simulink model "empirical_cell_twaice_balancing"  (R2024b)
settings: Solver=FixedStepAuto  StartTime=0.0  StopTime=inf  FixedStep=1  RelTol=1e-3
values from neighbouring files (symbols this model uses):
  act = 1    [RunMe_TWAICE_Cell_Model_Farasis_P75_75Ah_v8_1_3.m]
  lic_no = fin_convert(Prod_lic)    [RunMe_TWAICE_Cell_Model_Farasis_P75_75Ah_v8_1_3.m]
  Ts = 1    [RunMe_TWAICE_Cell_Model_Farasis_P75_75Ah_v8_1_3.m]
undefined symbols (not defined in the file or in its folder): DWORK0, DWORK1, DWORK10, DWORK11, DWORK12, DWORK13, DWORK14, DWORK15, DWORK16, DWORK17, DWORK18, DWORK19, DWORK2, DWORK20, DWORK22, DWORK23, DWORK24, DWORK25, DWORK26, DWORK27, DWORK28, DWORK29, DWORK3, DWORK30, DWORK31, DWORK32, DWORK33, DWORK34, DWORK35, DWORK36, DWORK4, DWORK5, DWORK6, DWORK7, DWORK8, DWORK9, SOHc_init, SOHr_init
libraries: fl_lib x73, nesl_utility x32, ee_lib x8
(part 1 of 4)
settings Model: PacingRate=60  Creator=CARSCH  LastModifiedBy=CARSCH
settings DebuggingCC: AlgebraicLoopMsg=none

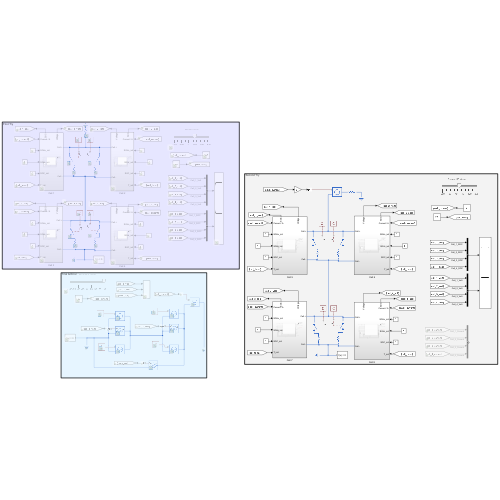
[thumbnail: Simulink's stored preview of the top-level diagram]
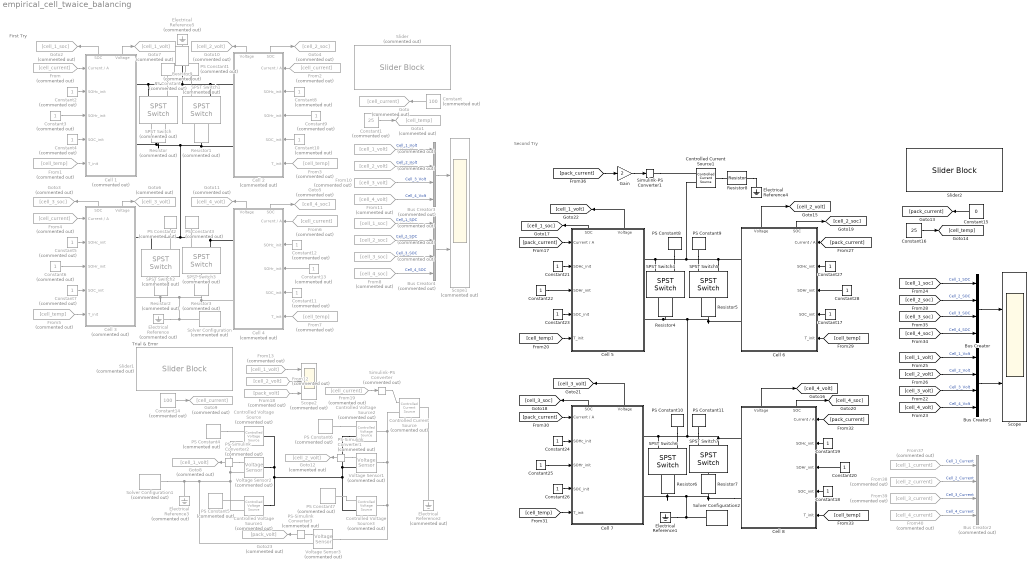
== system empirical_cell_twaice_balancing ==
  note: Trial & Error
  note: First Try
  note: Second Try
  Bus Creator : BusCreator  Inputs=4
  Bus Creator1 : BusCreator  Inputs=4
  Bus Creator2 : BusCreator  Commented=on  Inputs=4
  Bus Creator3 : BusCreator  Commented=on  Inputs=4
  Bus Creator4 : BusCreator  Commented=on  Inputs=4
  Cell 1 : Subsystem  Commented=on
      settings: PortSchema="{\"entries\":[{\"content\":{\"sides\":[{\"content\":{\"connectorIds\":[\"In1\",\"In2\",\"In3\",\"In4\",\"In5\"]},\"type\":\"ConnectorPlacement.EquallySpacedRectSide\",\"uuid\":\"39b6e759-d3e5-472a-9e81-7460229c4a62\"},{\"content\":{\"connectorIds\":[\"RConn1\",\"RConn2\"],\"side\":\"RIGHT\"},\"type\":\"ConnectorPlacement.EquallySpacedRectSide\",\"uuid\":\"f7fe5ccd-0242-4e3e-8253-e5b9b00b3385\"},{\"content\":{\"connectorIds\":[\"Out1\",\"Out2\"],\"side\":\"TOP\"},\"type\":\"ConnectorPlacement.EquallySpacedRectSide\",\"uuid\":\"deea17ee-3044-4fb2-b027-954681f0d31b\"}]},\"type\":\"ConnectorPlacement.EquallySpacedConnector\",\"uuid\":\"64bf650a-96e4-4191-8eb1-250115cba883\"}],\"packageUris\":[\"http://schema.mathworks.com/mf0/Connector/R2020b\"],\"version\":\"1.0\"}"
  Cell 2 : Subsystem  Commented=on
      settings: PortSchema="{\"entries\":[{\"content\":{\"sides\":[{\"content\":{\"connectorIds\":[\"In1\",\"In2\",\"In3\",\"In4\",\"In5\"]},\"type\":\"ConnectorPlacement.EquallySpacedRectSide\",\"uuid\":\"d8dd5e7d-9ddf-43d8-85ce-2acbe04dd73f\"},{\"content\":{\"connectorIds\":[\"RConn1\",\"RConn2\"],\"side\":\"RIGHT\"},\"type\":\"ConnectorPlacement.EquallySpacedRectSide\",\"uuid\":\"568b7dc0-f917-4967-8cc2-cd04b3e2240a\"},{\"content\":{\"connectorIds\":[\"Out1\",\"Out2\"],\"side\":\"TOP\"},\"type\":\"ConnectorPlacement.EquallySpacedRectSide\",\"uuid\":\"9700caac-c62d-4472-a735-ae999ee4f2e3\"}]},\"type\":\"ConnectorPlacement.EquallySpacedConnector\",\"uuid\":\"46beb2be-287e-49be-b6c7-ffcf4a8dc46d\"}],\"packageUris\":[\"http://schema.mathworks.com/mf0/Connector/R2020b\"],\"version\":\"1.0\"}"
  Cell 3 : Subsystem  Commented=on
      settings: PortSchema="{\"entries\":[{\"content\":{\"sides\":[{\"content\":{\"connectorIds\":[\"In1\",\"In2\",\"In3\",\"In4\",\"In5\"]},\"type\":\"ConnectorPlacement.EquallySpacedRectSide\",\"uuid\":\"d8dd5e7d-9ddf-43d8-85ce-2acbe04dd73f\"},{\"content\":{\"connectorIds\":[\"RConn1\",\"RConn2\"],\"side\":\"RIGHT\"},\"type\":\"ConnectorPlacement.EquallySpacedRectSide\",\"uuid\":\"568b7dc0-f917-4967-8cc2-cd04b3e2240a\"},{\"content\":{\"connectorIds\":[\"Out1\",\"Out2\"],\"side\":\"TOP\"},\"type\":\"ConnectorPlacement.EquallySpacedRectSide\",\"uuid\":\"9700caac-c62d-4472-a735-ae999ee4f2e3\"}]},\"type\":\"ConnectorPlacement.EquallySpacedConnector\",\"uuid\":\"46beb2be-287e-49be-b6c7-ffcf4a8dc46d\"}],\"packageUris\":[\"http://schema.mathworks.com/mf0/Connector/R2020b\"],\"version\":\"1.0\"}"
  Cell 4 : Subsystem  Commented=on
      settings: PortSchema="{\"entries\":[{\"content\":{\"sides\":[{\"content\":{\"connectorIds\":[\"In1\",\"In2\",\"In3\",\"In4\",\"In5\"]},\"type\":\"ConnectorPlacement.EquallySpacedRectSide\",\"uuid\":\"d8dd5e7d-9ddf-43d8-85ce-2acbe04dd73f\"},{\"content\":{\"connectorIds\":[\"RConn1\",\"RConn2\"],\"side\":\"RIGHT\"},\"type\":\"ConnectorPlacement.EquallySpacedRectSide\",\"uuid\":\"568b7dc0-f917-4967-8cc2-cd04b3e2240a\"},{\"content\":{\"connectorIds\":[\"Out1\",\"Out2\"],\"side\":\"TOP\"},\"type\":\"ConnectorPlacement.EquallySpacedRectSide\",\"uuid\":\"9700caac-c62d-4472-a735-ae999ee4f2e3\"}]},\"type\":\"ConnectorPlacement.EquallySpacedConnector\",\"uuid\":\"46beb2be-287e-49be-b6c7-ffcf4a8dc46d\"}],\"packageUris\":[\"http://schema.mathworks.com/mf0/Connector/R2020b\"],\"version\":\"1.0\"}"
  Cell 5 : Subsystem
      settings: PortSchema="{\"entries\":[{\"content\":{\"sides\":[{\"content\":{\"connectorIds\":[\"In1\",\"In2\",\"In3\",\"In4\",\"In5\"]},\"type\":\"ConnectorPlacement.EquallySpacedRectSide\",\"uuid\":\"39b6e759-d3e5-472a-9e81-7460229c4a62\"},{\"content\":{\"connectorIds\":[\"RConn1\",\"RConn2\"],\"side\":\"RIGHT\"},\"type\":\"ConnectorPlacement.EquallySpacedRectSide\",\"uuid\":\"f7fe5ccd-0242-4e3e-8253-e5b9b00b3385\"},{\"content\":{\"connectorIds\":[\"Out1\",\"Out2\"],\"side\":\"TOP\"},\"type\":\"ConnectorPlacement.EquallySpacedRectSide\",\"uuid\":\"deea17ee-3044-4fb2-b027-954681f0d31b\"}]},\"type\":\"ConnectorPlacement.EquallySpacedConnector\",\"uuid\":\"64bf650a-96e4-4191-8eb1-250115cba883\"}],\"packageUris\":[\"http://schema.mathworks.com/mf0/Connector/R2020b\"],\"version\":\"1.0\"}"
  Cell 6 : Subsystem
      settings: PortSchema="{\"entries\":[{\"content\":{\"sides\":[{\"content\":{\"connectorIds\":[\"In1\",\"In2\",\"In3\",\"In4\",\"In5\"]},\"type\":\"ConnectorPlacement.EquallySpacedRectSide\",\"uuid\":\"d8dd5e7d-9ddf-43d8-85ce-2acbe04dd73f\"},{\"content\":{\"connectorIds\":[\"RConn1\",\"RConn2\"],\"side\":\"RIGHT\"},\"type\":\"ConnectorPlacement.EquallySpacedRectSide\",\"uuid\":\"568b7dc0-f917-4967-8cc2-cd04b3e2240a\"},{\"content\":{\"connectorIds\":[\"Out1\",\"Out2\"],\"side\":\"TOP\"},\"type\":\"ConnectorPlacement.EquallySpacedRectSide\",\"uuid\":\"9700caac-c62d-4472-a735-ae999ee4f2e3\"}]},\"type\":\"ConnectorPlacement.EquallySpacedConnector\",\"uuid\":\"46beb2be-287e-49be-b6c7-ffcf4a8dc46d\"}],\"packageUris\":[\"http://schema.mathworks.com/mf0/Connector/R2020b\"],\"version\":\"1.0\"}"
  Cell 7 : Subsystem
      settings: PortSchema="{\"entries\":[{\"content\":{\"sides\":[{\"content\":{\"connectorIds\":[\"In1\",\"In2\",\"In3\",\"In4\",\"In5\"]},\"type\":\"ConnectorPlacement.EquallySpacedRectSide\",\"uuid\":\"d8dd5e7d-9ddf-43d8-85ce-2acbe04dd73f\"},{\"content\":{\"connectorIds\":[\"RConn1\",\"RConn2\"],\"side\":\"RIGHT\"},\"type\":\"ConnectorPlacement.EquallySpacedRectSide\",\"uuid\":\"568b7dc0-f917-4967-8cc2-cd04b3e2240a\"},{\"content\":{\"connectorIds\":[\"Out1\",\"Out2\"],\"side\":\"TOP\"},\"type\":\"ConnectorPlacement.EquallySpacedRectSide\",\"uuid\":\"9700caac-c62d-4472-a735-ae999ee4f2e3\"}]},\"type\":\"ConnectorPlacement.EquallySpacedConnector\",\"uuid\":\"46beb2be-287e-49be-b6c7-ffcf4a8dc46d\"}],\"packageUris\":[\"http://schema.mathworks.com/mf0/Connector/R2020b\"],\"version\":\"1.0\"}"
  Cell 8 : Subsystem
      settings: PortSchema="{\"entries\":[{\"content\":{\"sides\":[{\"content\":{\"connectorIds\":[\"In1\",\"In2\",\"In3\",\"In4\",\"In5\"]},\"type\":\"ConnectorPlacement.EquallySpacedRectSide\",\"uuid\":\"d8dd5e7d-9ddf-43d8-85ce-2acbe04dd73f\"},{\"content\":{\"connectorIds\":[\"RConn1\",\"RConn2\"],\"side\":\"RIGHT\"},\"type\":\"ConnectorPlacement.EquallySpacedRectSide\",\"uuid\":\"568b7dc0-f917-4967-8cc2-cd04b3e2240a\"},{\"content\":{\"connectorIds\":[\"Out1\",\"Out2\"],\"side\":\"TOP\"},\"type\":\"ConnectorPlacement.EquallySpacedRectSide\",\"uuid\":\"9700caac-c62d-4472-a735-ae999ee4f2e3\"}]},\"type\":\"ConnectorPlacement.EquallySpacedConnector\",\"uuid\":\"46beb2be-287e-49be-b6c7-ffcf4a8dc46d\"}],\"packageUris\":[\"http://schema.mathworks.com/mf0/Connector/R2020b\"],\"version\":\"1.0\"}"
  Constant : Constant  Commented=on  Value=100
  Constant1 : Constant  Commented=on  Value=25
  Constant{2..13} (12 alike) : Constant  Commented=on
  Constant14 : Constant  Commented=on  Value=100
  Constant15 : Constant  Value=0
  Constant16 : Constant  Value=25
  Constant{17..28} (12 alike) : Constant
  Controlled Current Source : fl_lib/Electrical/Electrical Sources/Controlled Current Source  Commented=on
  Controlled Current Source1 : fl_lib/Electrical/Electrical Sources/Controlled Current Source
  Controlled Voltage Source{,1..3} (4 alike) : fl_lib/Electrical/Electrical Sources/Controlled Voltage Source  Commented=on
  Electrical Reference{,2..3,5} (4 alike) : fl_lib/Electrical/Electrical Elements/Electrical Reference  Commented=on
  Electrical Reference1 : fl_lib/Electrical/Electrical Elements/Electrical Reference
  Electrical Reference4 : fl_lib/Electrical/Electrical Elements/Electrical Reference
  From{,2,4,6,19} (5 alike) : From  Commented=on  GotoTag=cell_current
  From{1,3,5,7} (4 alike) : From  Commented=on  GotoTag=cell_temp
  From10 : From  Commented=on  GotoTag=cell_3_volt
  From11 : From  Commented=on  GotoTag=cell_4_volt
  From12 : From  Commented=on  GotoTag=cell_2_volt
  From13 : From  Commented=on  GotoTag=cell_1_volt
  From14 : From  Commented=on  GotoTag=cell_1_soc
  From15 : From  Commented=on  GotoTag=cell_1_volt
  From16 : From  Commented=on  GotoTag=cell_2_volt
  From18 : From  Commented=on  GotoTag=pack_volt
  From21 : From  Commented=on  GotoTag=cell_2_soc
  From37 : From  Commented=on  GotoTag=cell_1_current
  From38 : From  Commented=on  GotoTag=cell_2_current
  From39 : From  Commented=on  GotoTag=cell_3_current
  From40 : From  Commented=on  GotoTag=cell_4_current
  From8 : From  Commented=on  GotoTag=cell_4_soc
  From9 : From  Commented=on  GotoTag=cell_3_soc
  Gain : Gain  Gain=2
  Goto : Goto  Commented=on  GotoTag=cell_current
  Goto1 : Goto  Commented=on  GotoTag=cell_temp
  Goto10 : Goto  Commented=on  GotoTag=cell_2_volt
  Goto11 : Goto  Commented=on  GotoTag=cell_4_volt
  Goto12 : Goto  Commented=on  GotoTag=cell_2_volt
  Goto2 : Goto  Commented=on  GotoTag=cell_1_soc
  Goto23 : Goto  Commented=on  GotoTag=pack_volt
  Goto3 : Goto  Commented=on  GotoTag=cell_3_soc
  Goto4 : Goto  Commented=on  GotoTag=cell_2_soc
  Goto5 : Goto  Commented=on  GotoTag=cell_4_soc
  Goto6 : Goto  Commented=on  GotoTag=cell_3_volt
  Goto7 : Goto  Commented=on  GotoTag=cell_1_volt
  Goto8 : Goto  Commented=on  GotoTag=cell_1_volt
  Goto9 : Goto  Commented=on  GotoTag=cell_current
  PS Constant{,1..3} (4 alike) : fl_lib/Physical Signals/Sources/PS Constant  Commented=on  constant=0
  PS Constant{8..11} (4 alike) : fl_lib/Physical Signals/Sources/PS Constant  constant=0
  PS Constant{4..7} (4 alike) : fl_lib/Physical Signals/Sources/PS Constant  Commented=on  constant=4.0 V
  PS-Simulink Converter1 : nesl_utility/PS-Simulink Converter  Commented=on  PhysicalDomain=network_engine_domain  SubClassName=ps_output  LeftPortType=input  RightPortType=output  PseudoPeriodic=off  Frequencies=[]  VectorFormat=inherit  Unit=inherit  AffineConversion=off
  PS-Simulink Converter2 : nesl_utility/PS-Simulink Converter  Commented=on  PhysicalDomain=network_engine_domain  SubClassName=ps_output  LeftPortType=input  RightPortType=output  PseudoPeriodic=off  Frequencies=[]  VectorFormat=inherit  Unit=inherit  AffineConversion=off
  PS-Simulink Converter3 : nesl_utility/PS-Simulink Converter  Commented=on  PhysicalDomain=network_engine_domain  SubClassName=ps_output  LeftPortType=input  RightPortType=output  PseudoPeriodic=off  Frequencies=[]  VectorFormat=inherit  Unit=inherit  AffineConversion=off
  Resistor{,1..3} (4 alike) : fl_lib/Electrical/Electrical Elements/Resistor  Commented=on  R=5 Ohm  i_specify=off  i_priority=None  i=0 A  i_nominal_specify=off  i_nominal_value=1  i_nominal_unit=A  v_specify=off  v_priority=None  v=0 V  v_nominal_specify=off  v_nominal_value=1  v_nominal_unit=V
  Resistor{4..7} (4 alike) : fl_lib/Electrical/Electrical Elements/Resistor  R=5 Ohm  i_specify=off  i_priority=None  i=0 A  i_nominal_specify=off  i_nominal_value=1  i_nominal_unit=A  v_specify=off  v_priority=None  v=0 V  v_nominal_specify=off  v_nominal_value=1  v_nominal_unit=V
  Resistor8 : fl_lib/Electrical/Electrical Elements/Resistor  R=100 Ohm  i_specify=off  i_priority=None  i=0 A  i_nominal_specify=off  i_nominal_value=1  i_nominal_unit=A  v_specify=off  v_priority=None  v=0 V  v_nominal_specify=off  v_nominal_value=1  v_nominal_unit=V
  Resistor9 : fl_lib/Electrical/Electrical Elements/Resistor  Commented=on  R=100 Ohm  i_specify=off  i_priority=None  i=0 A  i_nominal_specify=off  i_nominal_value=1  i_nominal_unit=A  v_specify=off  v_priority=None  v=0 V  v_nominal_specify=off  v_nominal_value=1  v_nominal_unit=V
  SPST Switch{,1..3} (4 alike) : ee_lib/Switches & Breakers/SPST Switch  Commented=on  R_closed=0.01 Ohm  G_open=1e-6 S  Threshold=0.5 V  Width=0 V  model_dynamics=0  t_on=1e-3 s  t_off=1e-3 s  initial_vT=0 V
      settings: InternalSimscapePortConfiguration="{\"Bottom\":[],\"Left\":[{\"id\":\"vT\",\"label\":\"vT\",\"type\":\"input\"},{\"id\":\"p\",\"label\":\"\",\"type\":\"foundation.electrical.electrical\"}],\"Right\":[{\"id\":\"n\",\"label\":\"\",\"type\":\"foundation.electrical.electrical\"}],\"Top\":[]}"
  SPST Switch{4..7} (4 alike) : ee_lib/Switches & Breakers/SPST Switch  R_closed=0.01 Ohm  G_open=1e-6 S  Threshold=0.5 V  Width=0 V  model_dynamics=0  t_on=1e-3 s  t_off=1e-3 s  initial_vT=0 V
      settings: InternalSimscapePortConfiguration="{\"Bottom\":[],\"Left\":[{\"id\":\"vT\",\"label\":\"vT\",\"type\":\"input\"},{\"id\":\"p\",\"label\":\"\",\"type\":\"foundation.electrical.electrical\"}],\"Right\":[{\"id\":\"n\",\"label\":\"\",\"type\":\"foundation.electrical.electrical\"}],\"Top\":[]}"
  Scope : Scope  NumInputPorts=2
  Scope1 : Scope  Commented=on  NumInputPorts=2
  Scope2 : Scope  Commented=on  NumInputPorts=3
  Simulink-PS Converter : nesl_utility/Simulink-PS Converter  Commented=on  PhysicalDomain=network_engine_domain  SubClassName=ps_input  LeftPortType=input  RightPortType=output  PseudoPeriodic=off  Frequencies=[]  NoiseDistribution=none  NoiseParameters=[]  Unit=1  AffineConversion=off  FilteringAndDerivatives=provide  SimscapeFilterOrder=1  InputFilterTimeConstant=0.001  UdotUserProvided=0
  Simulink-PS Converter1 : nesl_utility/Simulink-PS Converter  PhysicalDomain=network_engine_domain  SubClassName=ps_input  LeftPortType=input  RightPortType=output  PseudoPeriodic=off  Frequencies=[]  NoiseDistribution=none  NoiseParameters=[]  Unit=1  AffineConversion=off  FilteringAndDerivatives=provide  SimscapeFilterOrder=1  InputFilterTimeConstant=0.001  UdotUserProvided=0
  Slider : SliderBlock  Commented=on  ScaleMin=-200  ScaleMax=300
  Slider1 : SliderBlock  Commented=on  ScaleMin=-100
  Slider2 : SliderBlock  ScaleMin=-200  ScaleMax=200
  Solver Configuration : nesl_utility/Solver Configuration  Commented=on  PhysicalDomain=network_engine_domain  SubClassName=solver  LeftPortType=input  RightPortType=generic  Tones=[]  Harmonics=[]  SimulateNoise=off  Profile=off  UseLocalSampling=off  EnableSwitchedLinearOptims=on  FrequencyDomain=off  UseCCode=off  RelTol=0.001  AbsTol=0.001  MinStep=1e-09  ToWorkspace=off  RevertToSquareIcSolve=off  NumHomotopyIterations=100  PhasorMode=off  PhasorModeNumHarmonics=1  ConsistencySolver=NEWTON_XTOL_AFTER_FTOL  IndexReductionMethod=DerivativeReplacement  DoDC=on  ResidualTolerance=1e-09  ConsistencyTolSource=GLOBAL  ConsistencyAbsTol=0.001  ConsistencyRelTol=0.001  ConsistencyTolFactor=0.001  UseLocalSolver=off  LocalSolverChoice=NE_BACKWARD_EULER_ADVANCER  ResolveIndetEquations=on  FunctionEvalNumThread=1  LocalSolverSampleTime=0.001  DoFixedCost=off  MaxNonlinIter=3  MaxModeIter=2  ComputeImpulses=off  ImpulseIterations=2  LinearAlgebra=auto  LinearAlgebraNumThread=0  EquationFormulation=NE_TIME_EF  DelaysMemoryBudget=1024  AutomaticFiltering=on  FilteringTimeConstant=0.001  PartitionStorageMethod=AS_NEEDED  PartitionMemoryBudget=1024  PartitionMethod=ROBUST  MultibodyUseLocalSolver=off  MultibodyLocalSolverChoice=ODE1  MultibodyLocalSolverSampleTime=0.001
  Solver Configuration1 : nesl_utility/Solver Configuration  Commented=on  PhysicalDomain=network_engine_domain  SubClassName=solver  LeftPortType=input  RightPortType=generic  Tones=[]  Harmonics=[]  SimulateNoise=off  Profile=off  UseLocalSampling=off  EnableSwitchedLinearOptims=on  FrequencyDomain=off  UseCCode=off  RelTol=0.001  AbsTol=0.001  MinStep=1e-09  ToWorkspace=off  RevertToSquareIcSolve=off  NumHomotopyIterations=100  PhasorMode=off  PhasorModeNumHarmonics=1  ConsistencySolver=NEWTON_XTOL_AFTER_FTOL  IndexReductionMethod=DerivativeReplacement  DoDC=off  ResidualTolerance=1e-09  ConsistencyTolSource=GLOBAL  ConsistencyAbsTol=0.001  ConsistencyRelTol=0.001  ConsistencyTolFactor=0.001  UseLocalSolver=off  LocalSolverChoice=NE_BACKWARD_EULER_ADVANCER  ResolveIndetEquations=on  FunctionEvalNumThread=1  LocalSolverSampleTime=0.001  DoFixedCost=off  MaxNonlinIter=3  MaxModeIter=2  ComputeImpulses=off  ImpulseIterations=2  LinearAlgebra=auto  LinearAlgebraNumThread=0  EquationFormulation=NE_TIME_EF  DelaysMemoryBudget=1024  AutomaticFiltering=on  FilteringTimeConstant=0.001  PartitionStorageMethod=AS_NEEDED  PartitionMemoryBudget=1024  PartitionMethod=ROBUST  MultibodyUseLocalSolver=off  MultibodyLocalSolverChoice=ODE1  MultibodyLocalSolverSampleTime=0.001
  Solver Configuration2 : nesl_utility/Solver Configuration  PhysicalDomain=network_engine_domain  SubClassName=solver  LeftPortType=input  RightPortType=generic  Tones=[]  Harmonics=[]  SimulateNoise=off  Profile=off  UseLocalSampling=off  EnableSwitchedLinearOptims=on  FrequencyDomain=off  UseCCode=off  RelTol=0.001  AbsTol=0.001  MinStep=1e-09  ToWorkspace=off  RevertToSquareIcSolve=off  NumHomotopyIterations=100  PhasorMode=off  PhasorModeNumHarmonics=1  ConsistencySolver=NEWTON_XTOL_AFTER_FTOL  IndexReductionMethod=DerivativeReplacement  DoDC=on  ResidualTolerance=1e-09  ConsistencyTolSource=GLOBAL  ConsistencyAbsTol=0.001  ConsistencyRelTol=0.001  ConsistencyTolFactor=0.001  UseLocalSolver=off  LocalSolverChoice=NE_BACKWARD_EULER_ADVANCER  ResolveIndetEquations=on  FunctionEvalNumThread=1  LocalSolverSampleTime=0.001  DoFixedCost=off  MaxNonlinIter=3  MaxModeIter=2  ComputeImpulses=off  ImpulseIterations=2  LinearAlgebra=auto  LinearAlgebraNumThread=0  EquationFormulation=NE_TIME_EF  DelaysMemoryBudget=1024  AutomaticFiltering=on  FilteringTimeConstant=0.001  PartitionStorageMethod=AS_NEEDED  PartitionMemoryBudget=1024  PartitionMethod=ROBUST  MultibodyUseLocalSolver=off  MultibodyLocalSolverChoice=ODE1  MultibodyLocalSolverSampleTime=0.001
  Voltage Sensor1 : fl_lib/Electrical/Electrical Sensors/Voltage Sensor  Commented=on
  Voltage Sensor2 : fl_lib/Electrical/Electrical Sensors/Voltage Sensor  Commented=on
  Voltage Sensor3 : fl_lib/Electrical/Electrical Sensors/Voltage Sensor  Commented=on
  wires:
  From/1 -> Cell 1/1("Current / A ")
  Constant/1 -> Goto/1
  Constant1/1 -> Goto1/1
  From1/1 -> Cell 1/5(T_init)
  From2/1 -> Cell 2/1("Current / A ")
  From3/1 -> Cell 2/5(T_init)
  From6/1 -> Cell 4/1("Current / A ")
  From4/1 -> Cell 3/1("Current / A ")
  From7/1 -> Cell 4/5(T_init)
  From5/1 -> Cell 3/5(T_init)
  Constant2/1 -> Cell 1/2(SOHc_init)
  Constant3/1 -> Cell 1/3(SOHr_init)
  Constant4/1 -> Cell 1/4(SOC_init)
  Constant7/1 -> Cell 3/4(SOC_init)
  Constant5/1 -> Cell 3/2(SOHc_init)
  Constant6/1 -> Cell 3/3(SOHr_init)
  Constant8/1 -> Cell 2/2(SOHc_init)
  Constant9/1 -> Cell 2/3(SOHr_init)
  Constant10/1 -> Cell 2/4(SOC_init)
  Constant12/1 -> Cell 4/2(SOHc_init)
  Constant11/1 -> Cell 4/4(SOC_init)
  Constant13/1 -> Cell 4/3(SOHr_init)
  Cell 3/1(SOC) -> Goto3/1
  PS-Simulink Converter2/1 -> Goto8/1
  From13/1 -> Scope2/1
  Constant14/1 -> Goto9/1
  From19/1 -> Simulink-PS Converter/1
  Cell 2/1(SOC) -> Goto4/1
  Cell 1/1(SOC) -> Goto2/1
  From16/1 -> Bus Creator3/2  "Cell_2_Volt"
  From15/1 -> Bus Creator3/1  "Cell_1_Volt"
  Cell 1/2(Voltage) -> Goto7/1
  Cell 2/2(Voltage) -> Goto10/1
  Cell 4/1(SOC) -> Goto5/1
  Cell 3/2(Voltage) -> Goto6/1
  Cell 4/2(Voltage) -> Goto11/1
  From21/1 -> Bus Creator4/2  "Cell_2_SOC"
  From14/1 -> Bus Creator4/1  "Cell_1_SOC"
  From8/1 -> Bus Creator4/4  "Cell_4_SOC"
  From9/1 -> Bus Creator4/3  "Cell_3_SOC"
  From10/1 -> Bus Creator3/3  "Cell_3_Volt"
  From11/1 -> Bus Creator3/4  "Cell_4_Volt"
  PS-Simulink Converter1/1 -> Goto12/1
  From18/1 -> Scope2/3
  From12/1 -> Scope2/2
  [cell_1_soc] -> Bus Creator/1  "Cell_1_SOC"
  [cell_3_volt] -> Bus Creator1/3  "Cell_3_Volt"
  Cell 7/1(SOC) -> [cell_3_soc]
  Cell 5/1(SOC) -> [cell_1_soc]
  Cell 8/2(Voltage) -> [cell_4_volt]
  Cell 6/1(SOC) -> [cell_2_soc]
  [cell_4_volt] -> Bus Creator1/4  "Cell_4_Volt"
  Cell 7/2(Voltage) -> [cell_3_volt]
  Constant23/1 -> Cell 5/4(SOC_init)
  Constant22/1 -> Cell 5/3(SOHr_init)
  Cell 8/1(SOC) -> [cell_4_soc]
  Constant27/1 -> Cell 6/2(SOHc_init)
  Constant18/1 -> Cell 8/4(SOC_init)
  Constant25/1 -> Cell 7/3(SOHr_init)
  Constant20/1 -> Cell 8/3(SOHr_init)
  [cell_3_soc] -> Bus Creator/3  "Cell_3_SOC"
  Constant19/1 -> Cell 8/2(SOHc_init)
  [cell_temp] -> Cell 8/5(T_init)
  Cell 5/2(Voltage) -> [cell_1_volt]
  Cell 6/2(Voltage) -> [cell_2_volt]
  [pack_current] -> Cell 7/1("Current / A ")
  Constant17/1 -> Cell 6/4(SOC_init)
  [cell_2_soc] -> Bus Creator/2  "Cell_2_SOC"
  Constant16/1 -> [cell_temp]
  [cell_4_soc] -> Bus Creator/4  "Cell_4_SOC"
  [pack_current] -> Cell 6/1("Current / A ")
  [cell_temp] -> Cell 6/5(T_init)
  [pack_current] -> Cell 8/1("Current / A ")
  [cell_1_volt] -> Bus Creator1/1  "Cell_1_Volt"
  [cell_2_volt] -> Bus Creator1/2  "Cell_2_Volt"
  [pack_current] -> Cell 5/1("Current / A ")
  Constant26/1 -> Cell 7/4(SOC_init)
  Constant21/1 -> Cell 5/2(SOHc_init)
  Constant24/1 -> Cell 7/2(SOHc_init)
  Constant15/1 -> [pack_current]
  Constant28/1 -> Cell 6/3(SOHr_init)
  [cell_temp] -> Cell 5/5(T_init)
  [cell_temp] -> Cell 7/5(T_init)
  PS-Simulink Converter3/1 -> Goto23/1
  [pack_current] -> Gain/1
  Gain/1 -> Simulink-PS Converter1/1
  From40/1 -> Bus Creator2/4  "Cell_4_Current"
  From38/1 -> Bus Creator2/2  "Cell_2_Current"
  From39/1 -> Bus Creator2/3  "Cell_3_Current"
  From37/1 -> Bus Creator2/1  "Cell_1_Current"
  Bus Creator/1 -> Scope/1
  Bus Creator1/1 -> Scope/2
  Bus Creator3/1 -> Scope1/1
  Bus Creator4/1 -> Scope1/2
  connections:
  Resistor/RConn1 -- Cell 1/RConn2 -- Cell 3/RConn1 -- SPST Switch2/LConn2 -- SPST Switch3/LConn2 -- Cell 4/RConn1 -- Cell 2/RConn2 -- Resistor1/RConn1
  SPST Switch/RConn1 -- Resistor/LConn1
  Resistor1/LConn1 -- SPST Switch1/RConn1
  Resistor2/RConn1 -- Cell 3/RConn2 -- Solver Configuration/RConn1 -- Electrical Reference/LConn1 -- Resistor3/RConn1 -- Cell 4/RConn2
  Resistor2/LConn1 -- SPST Switch2/RConn1
  Resistor3/LConn1 -- SPST Switch3/RConn1
  SPST Switch/LConn2 -- Cell 1/RConn1 -- Resistor9/LConn1 -- Cell 2/RConn1 -- SPST Switch1/LConn2
  PS Constant/RConn1 -- SPST Switch/LConn1
  PS Constant1/RConn1 -- SPST Switch1/LConn1
  PS Constant2/RConn1 -- SPST Switch2/LConn1
  PS Constant3/RConn1 -- SPST Switch3/LConn1
  Controlled Voltage Source2/RConn2 -- Controlled Voltage Source1/LConn1 -- Controlled Voltage Source/LConn1 -- Voltage Sensor2/LConn1 -- Controlled Voltage Source3/RConn2 -- Voltage Sensor1/RConn2
  PS Constant4/RConn1 -- Controlled Voltage Source/RConn1
  Simulink-PS Converter/RConn1 -- Controlled Current Source/RConn1
  Electrical Reference3/LConn1 -- Voltage Sensor3/RConn2 -- Controlled Voltage Source1/RConn2 -- Voltage Sensor2/RConn2 -- Controlled Voltage Source/RConn2 -- Solver Configuration1/RConn1
  Electrical Reference2/LConn1 -- Controlled Current Source/LConn1
  PS-Simulink Converter2/LConn1 -- Voltage Sensor2/RConn1
  PS Constant5/RConn1 -- Controlled Voltage Source1/RConn1
  Voltage Sensor1/LConn1 -- Voltage Sensor3/LConn1 -- Controlled Voltage Source3/LConn1 -- Controlled Current Source/RConn2 -- Controlled Voltage Source2/LConn1
  PS-Simulink Converter1/LConn1 -- Voltage Sensor1/RConn1
  PS Constant7/RConn1 -- Controlled Voltage Source3/RConn1
  PS Constant6/RConn1 -- Controlled Voltage Source2/RConn1
  Resistor5/RConn1 -- Cell 6/RConn2 -- Cell 7/RConn1 -- SPST Switch6/LConn2 -- SPST Switch7/LConn2 -- Cell 8/RConn1 -- Cell 5/RConn2 -- Resistor4/RConn1
  Cell 8/RConn2 -- Solver Configuration2/RConn1 -- Electrical Reference1/LConn1 -- Cell 7/RConn2 -- Resistor6/RConn1 -- Resistor7/RConn1
  SPST Switch5/LConn2 -- Controlled Current Source1/RConn2 -- Cell 5/RConn1 -- SPST Switch4/LConn2 -- Cell 6/RConn1
  Resistor5/LConn1 -- SPST Switch5/RConn1
  Resistor7/LConn1 -- SPST Switch7/RConn1
  PS Constant11/RConn1 -- SPST Switch7/LConn1
  SPST Switch4/RConn1 -- Resistor4/LConn1
  PS Constant8/RConn1 -- SPST Switch4/LConn1
  PS Constant9/RConn1 -- SPST Switch5/LConn1
  PS Constant10/RConn1 -- SPST Switch6/LConn1
  Resistor6/LConn1 -- SPST Switch6/RConn1
  PS-Simulink Converter3/LConn1 -- Voltage Sensor3/RConn1
  Controlled Current Source1/LConn1 -- Resistor8/LConn1
  Simulink-PS Converter1/RConn1 -- Controlled Current Source1/RConn1
  Resistor8/RConn1 -- Electrical Reference4/LConn1
  Electrical Reference5/LConn1 -- Resistor9/RConn1

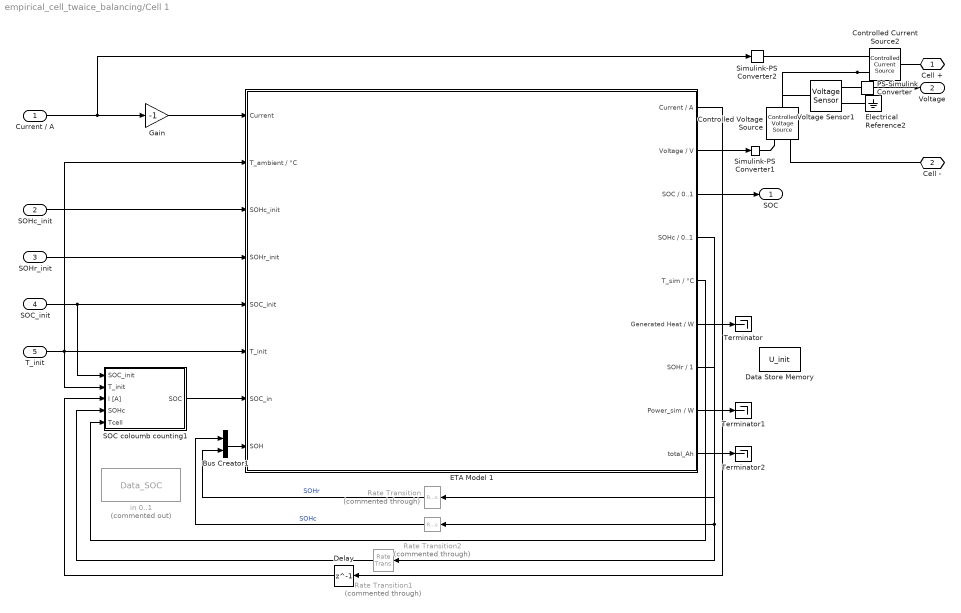
== system empirical_cell_twaice_balancing/Cell 1 ==
  "Current / A " : Inport  OutDataTypeStr=double  PortDimensions=1
  SOHc_init : Inport  Port=2
  SOHr_init : Inport  Port=3
  SOC_init : Inport  Port=4
  T_init : Inport  Port=5
  Bus Creator1 : BusCreator  Inputs=2
  Controlled Current Source2 : fl_lib/Electrical/Electrical Sources/Controlled Current Source
  Controlled Voltage Source : fl_lib/Electrical/Electrical Sources/Controlled Voltage Source
  Data Store Memory : DataStoreMemory  DataStoreName=U_init  WriteAfterWriteMsg=warning  ShowAdditionalParam=off
  Delay : Delay  DelayLength=1
  ETA Model 1 : Subsystem  mask{sfcnParam1=Ts, sfcnParam2=act, sfcnParam3=lic_no}
      mask prompts: sfcnParam1 "Ts:"; sfcnParam2 "act:"; sfcnParam3 "lic_no:"
      mask help: Simulink:masks:GenSFuncDesc_MD
      mask Help: eval('feval(''rtwprivate'',''rtwhelpview'',''rtw_sfcn_block'')');
  Electrical Reference2 : fl_lib/Electrical/Electrical Elements/Electrical Reference
  Gain : Gain  Gain=-1
  PS-Simulink Converter : nesl_utility/PS-Simulink Converter  PhysicalDomain=network_engine_domain  SubClassName=ps_output  LeftPortType=input  RightPortType=output  PseudoPeriodic=off  Frequencies=[]  VectorFormat=inherit  Unit=inherit  AffineConversion=on
  Rate Transition : RateTransition  Commented=through  InitialCondition=SOHr_init
  Rate Transition1 : RateTransition  Commented=through  InitialCondition=SOHc_init
  Rate Transition2 : RateTransition  Commented=through  InitialCondition=SOHc_init
  SOC coloumb counting1 : Subsystem  mask{sfcnParam1=Ts}
      mask prompts: sfcnParam1 "Ts:"
      mask help: Simulink:masks:GenSFuncDesc_MD
      mask Help: eval('feval(''rtwprivate'',''rtwhelpview'',''rtw_sfcn_block'')');
  Simulink-PS Converter1 : nesl_utility/Simulink-PS Converter  PhysicalDomain=network_engine_domain  SubClassName=ps_input  LeftPortType=input  RightPortType=output  PseudoPeriodic=off  Frequencies=[]  NoiseDistribution=none  NoiseParameters=[]  Unit=1  AffineConversion=on  FilteringAndDerivatives=provide  SimscapeFilterOrder=1  InputFilterTimeConstant=0.001  UdotUserProvided=0
  Simulink-PS Converter2 : nesl_utility/Simulink-PS Converter  PhysicalDomain=network_engine_domain  SubClassName=ps_input  LeftPortType=input  RightPortType=output  PseudoPeriodic=off  Frequencies=[]  NoiseDistribution=none  NoiseParameters=[]  Unit=1  AffineConversion=on  FilteringAndDerivatives=provide  SimscapeFilterOrder=1  InputFilterTimeConstant=0.001  UdotUserProvided=0
  Terminator : Terminator
  Terminator1 : Terminator
  Terminator2 : Terminator
  Voltage Sensor1 : fl_lib/Electrical/Electrical Sensors/Voltage Sensor
  in 0..1 : FromWorkspace  Commented=on  VariableName=Data_SOC  SampleTime=Ts  OutputAfterFinalValue=Setting to zero
  Cell + : PMIOPort  Side=Right
  Cell - : PMIOPort  Port=2  Side=Right
  SOC : Outport
  Voltage : Outport  Port=2
  wires:
  Rate Transition/1 -> Bus Creator1/2  "SOHr"
  T_init/1 -> ETA Model 1/2(T_ambient / °C), SOC coloumb counting1/2(T_init), ETA Model 1/6(T_init)
  ETA Model 1/3(SOC / 0..1) -> SOC/1
  ETA Model 1/4(SOHc / 0..1) -> Rate Transition2/1, Rate Transition1/1
  SOC_init/1 -> SOC coloumb counting1/1(SOC_init), ETA Model 1/5(SOC_init)
  Rate Transition1/1 -> SOC coloumb counting1/4(SOHc)
  SOHc_init/1 -> ETA Model 1/3(SOHc_init)
  ETA Model 1/9(total_Ah) -> Terminator2/1
  ETA Model 1/7(SOHr / 1) -> Rate Transition/1
  ETA Model 1/1(Current / A) -> Delay/1
  ETA Model 1/5(T_sim / °C) -> SOC coloumb counting1/5(Tcell)
  SOC coloumb counting1/1(SOC) -> ETA Model 1/7(SOC_in)
  ETA Model 1/8(Power_sim / W) -> Terminator1/1
  Delay/1 -> SOC coloumb counting1/3(I [A])
  Bus Creator1/1 -> ETA Model 1/8(SOH)
  Rate Transition2/1 -> Bus Creator1/1  "SOHc"
  SOHr_init/1 -> ETA Model 1/4(SOHr_init)
  ETA Model 1/6(Generated Heat / W) -> Terminator/1
  Gain/1 -> ETA Model 1/1("Current ")
  ETA Model 1/2(Voltage / V) -> Simulink-PS Converter1/1
  "Current / A "/1 -> Simulink-PS Converter2/1, Gain/1
  PS-Simulink Converter/1 -> Voltage/1
  connections:
  Controlled Current Source2/RConn2 -- Voltage Sensor1/LConn1 -- Controlled Voltage Source/LConn1
  Simulink-PS Converter1/RConn1 -- Controlled Voltage Source/RConn1
  Controlled Current Source2/RConn1 -- Simulink-PS Converter2/RConn1
  PS-Simulink Converter/LConn1 -- Voltage Sensor1/RConn1
  Controlled Voltage Source/RConn2 -- Cell -/RConn1
  Cell +/RConn1 -- Controlled Current Source2/LConn1
  Electrical Reference2/LConn1 -- Voltage Sensor1/RConn2

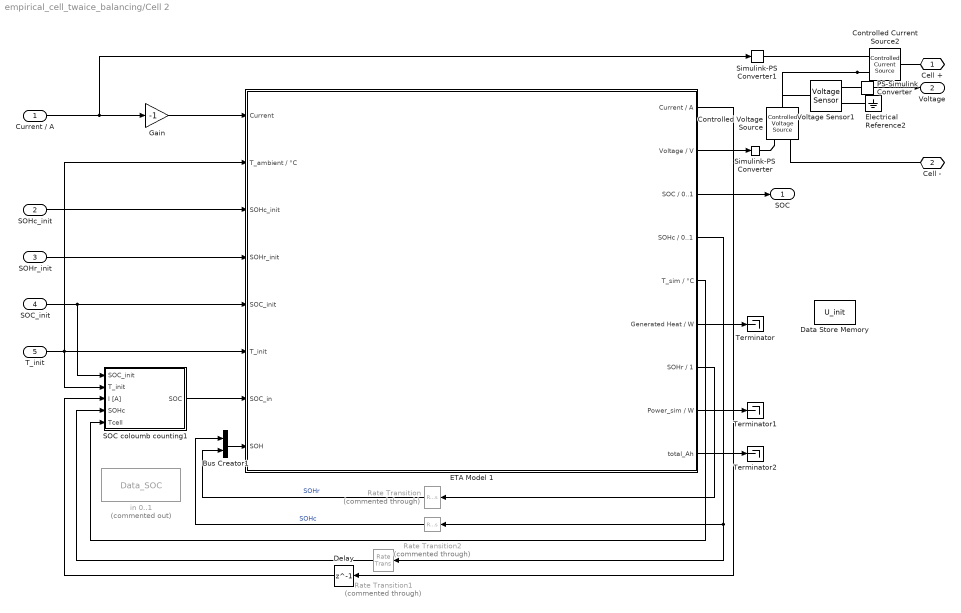
== system empirical_cell_twaice_balancing/Cell 2 ==
  "Current / A " : Inport  OutDataTypeStr=double  PortDimensions=1
  SOHc_init : Inport  Port=2
  SOHr_init : Inport  Port=3
  SOC_init : Inport  Port=4
  T_init : Inport  Port=5
  Bus Creator1 : BusCreator  Inputs=2
  Controlled Current Source2 : fl_lib/Electrical/Electrical Sources/Controlled Current Source
  Controlled Voltage Source : fl_lib/Electrical/Electrical Sources/Controlled Voltage Source
  Data Store Memory : DataStoreMemory  DataStoreName=U_init  WriteAfterWriteMsg=warning  ShowAdditionalParam=off
  Delay : Delay  DelayLength=1
  ETA Model 1 : Subsystem  mask{sfcnParam1=Ts, sfcnParam2=act, sfcnParam3=lic_no}
      mask prompts: sfcnParam1 "Ts:"; sfcnParam2 "act:"; sfcnParam3 "lic_no:"
      mask help: Simulink:masks:GenSFuncDesc_MD
      mask Help: eval('feval(''rtwprivate'',''rtwhelpview'',''rtw_sfcn_block'')');
  Electrical Reference2 : fl_lib/Electrical/Electrical Elements/Electrical Reference
  Gain : Gain  Gain=-1
  PS-Simulink Converter : nesl_utility/PS-Simulink Converter  PhysicalDomain=network_engine_domain  SubClassName=ps_output  LeftPortType=input  RightPortType=output  PseudoPeriodic=off  Frequencies=[]  VectorFormat=inherit  Unit=inherit  AffineConversion=on
  Rate Transition : RateTransition  Commented=through  InitialCondition=SOHr_init
  Rate Transition1 : RateTransition  Commented=through  InitialCondition=SOHc_init
  Rate Transition2 : RateTransition  Commented=through  InitialCondition=SOHc_init
  SOC coloumb counting1 : Subsystem  mask{sfcnParam1=Ts}
      mask prompts: sfcnParam1 "Ts:"
      mask help: Simulink:masks:GenSFuncDesc_MD
      mask Help: eval('feval(''rtwprivate'',''rtwhelpview'',''rtw_sfcn_block'')');
  Simulink-PS Converter : nesl_utility/Simulink-PS Converter  PhysicalDomain=network_engine_domain  SubClassName=ps_input  LeftPortType=input  RightPortType=output  PseudoPeriodic=off  Frequencies=[]  NoiseDistribution=none  NoiseParameters=[]  Unit=1  AffineConversion=on  FilteringAndDerivatives=provide  SimscapeFilterOrder=1  InputFilterTimeConstant=0.001  UdotUserProvided=0
  Simulink-PS Converter1 : nesl_utility/Simulink-PS Converter  PhysicalDomain=network_engine_domain  SubClassName=ps_input  LeftPortType=input  RightPortType=output  PseudoPeriodic=off  Frequencies=[]  NoiseDistribution=none  NoiseParameters=[]  Unit=1  AffineConversion=on  FilteringAndDerivatives=provide  SimscapeFilterOrder=1  InputFilterTimeConstant=0.001  UdotUserProvided=0
  Terminator : Terminator
  Terminator1 : Terminator
  Terminator2 : Terminator
  Voltage Sensor1 : fl_lib/Electrical/Electrical Sensors/Voltage Sensor
  in 0..1 : FromWorkspace  Commented=on  VariableName=Data_SOC  SampleTime=Ts  OutputAfterFinalValue=Setting to zero
  Cell + : PMIOPort  Side=Right
  Cell - : PMIOPort  Port=2  Side=Right
  SOC : Outport
  Voltage : Outport  Port=2
  wires:
  Rate Transition/1 -> Bus Creator1/2  "SOHr"
  T_init/1 -> ETA Model 1/2(T_ambient / °C), SOC coloumb counting1/2(T_init), ETA Model 1/6(T_init)
  ETA Model 1/4(SOHc / 0..1) -> Rate Transition2/1, Rate Transition1/1
  SOC_init/1 -> SOC coloumb counting1/1(SOC_init), ETA Model 1/5(SOC_init)
  Rate Transition1/1 -> SOC coloumb counting1/4(SOHc)
  SOHc_init/1 -> ETA Model 1/3(SOHc_init)
  ETA Model 1/9(total_Ah) -> Terminator2/1
  ETA Model 1/7(SOHr / 1) -> Rate Transition/1
  ETA Model 1/1(Current / A) -> Delay/1
  ETA Model 1/5(T_sim / °C) -> SOC coloumb counting1/5(Tcell)
  SOC coloumb counting1/1(SOC) -> ETA Model 1/7(SOC_in)
  ETA Model 1/8(Power_sim / W) -> Terminator1/1
  Delay/1 -> SOC coloumb counting1/3(I [A])
  Bus Creator1/1 -> ETA Model 1/8(SOH)
  Rate Transition2/1 -> Bus Creator1/1  "SOHc"
  "Current / A "/1 -> Simulink-PS Converter1/1, Gain/1
  SOHr_init/1 -> ETA Model 1/4(SOHr_init)
  ETA Model 1/6(Generated Heat / W) -> Terminator/1
  ETA Model 1/2(Voltage / V) -> Simulink-PS Converter/1
  Gain/1 -> ETA Model 1/1("Current ")
  ETA Model 1/3(SOC / 0..1) -> SOC/1
  PS-Simulink Converter/1 -> Voltage/1
  connections:
  Controlled Current Source2/RConn2 -- Voltage Sensor1/LConn1 -- Controlled Voltage Source/LConn1
  Controlled Current Source2/RConn1 -- Simulink-PS Converter1/RConn1
  Controlled Voltage Source/RConn2 -- Cell -/RConn1
  Cell +/RConn1 -- Controlled Current Source2/LConn1
  Electrical Reference2/LConn1 -- Voltage Sensor1/RConn2
  Simulink-PS Converter/RConn1 -- Controlled Voltage Source/RConn1
  PS-Simulink Converter/LConn1 -- Voltage Sensor1/RConn1

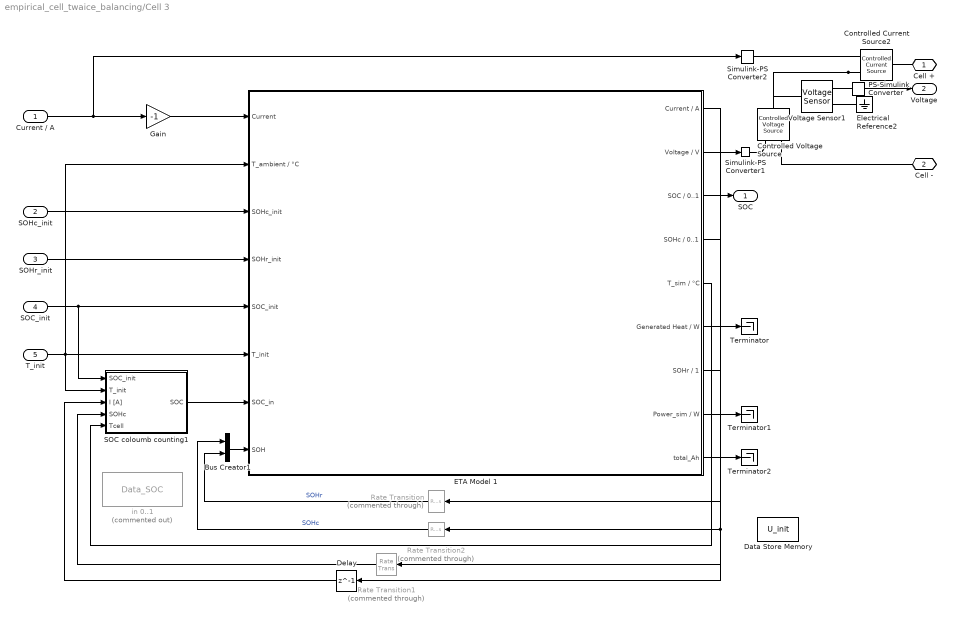
== system empirical_cell_twaice_balancing/Cell 3 ==
  "Current / A " : Inport  OutDataTypeStr=double  PortDimensions=1
  SOHc_init : Inport  Port=2
  SOHr_init : Inport  Port=3
  SOC_init : Inport  Port=4
  T_init : Inport  Port=5
  Bus Creator1 : BusCreator  Inputs=2
  Controlled Current Source2 : fl_lib/Electrical/Electrical Sources/Controlled Current Source
  Controlled Voltage Source : fl_lib/Electrical/Electrical Sources/Controlled Voltage Source
  Data Store Memory : DataStoreMemory  DataStoreName=U_init  WriteAfterWriteMsg=warning  ShowAdditionalParam=off
  Delay : Delay  DelayLength=1
  ETA Model 1 : Subsystem  mask{sfcnParam1=Ts, sfcnParam2=act, sfcnParam3=lic_no}
      mask prompts: sfcnParam1 "Ts:"; sfcnParam2 "act:"; sfcnParam3 "lic_no:"
      mask help: Simulink:masks:GenSFuncDesc_MD
      mask Help: eval('feval(''rtwprivate'',''rtwhelpview'',''rtw_sfcn_block'')');
  Electrical Reference2 : fl_lib/Electrical/Electrical Elements/Electrical Reference
  Gain : Gain  Gain=-1
  PS-Simulink Converter : nesl_utility/PS-Simulink Converter  PhysicalDomain=network_engine_domain  SubClassName=ps_output  LeftPortType=input  RightPortType=output  PseudoPeriodic=off  Frequencies=[]  VectorFormat=inherit  Unit=inherit  AffineConversion=on
  Rate Transition : RateTransition  Commented=through  InitialCondition=SOHr_init
  Rate Transition1 : RateTransition  Commented=through  InitialCondition=SOHc_init
  Rate Transition2 : RateTransition  Commented=through  InitialCondition=SOHc_init
  SOC coloumb counting1 : Subsystem  mask{sfcnParam1=Ts}
      mask prompts: sfcnParam1 "Ts:"
      mask help: Simulink:masks:GenSFuncDesc_MD
      mask Help: eval('feval(''rtwprivate'',''rtwhelpview'',''rtw_sfcn_block'')');
  Simulink-PS Converter1 : nesl_utility/Simulink-PS Converter  PhysicalDomain=network_engine_domain  SubClassName=ps_input  LeftPortType=input  RightPortType=output  PseudoPeriodic=off  Frequencies=[]  NoiseDistribution=none  NoiseParameters=[]  Unit=1  AffineConversion=on  FilteringAndDerivatives=provide  SimscapeFilterOrder=1  InputFilterTimeConstant=0.001  UdotUserProvided=0
  Simulink-PS Converter2 : nesl_utility/Simulink-PS Converter  PhysicalDomain=network_engine_domain  SubClassName=ps_input  LeftPortType=input  RightPortType=output  PseudoPeriodic=off  Frequencies=[]  NoiseDistribution=none  NoiseParameters=[]  Unit=1  AffineConversion=on  FilteringAndDerivatives=provide  SimscapeFilterOrder=1  InputFilterTimeConstant=0.001  UdotUserProvided=0
  Terminator : Terminator
  Terminator1 : Terminator
  Terminator2 : Terminator
  Voltage Sensor1 : fl_lib/Electrical/Electrical Sensors/Voltage Sensor
  in 0..1 : FromWorkspace  Commented=on  VariableName=Data_SOC  SampleTime=Ts  OutputAfterFinalValue=Setting to zero
  Cell + : PMIOPort  Side=Right
  Cell - : PMIOPort  Port=2  Side=Right
  SOC : Outport
  Voltage : Outport  Port=2
  wires:
  Rate Transition/1 -> Bus Creator1/2  "SOHr"
  T_init/1 -> ETA Model 1/2(T_ambient / °C), SOC coloumb counting1/2(T_init), ETA Model 1/6(T_init)
  ETA Model 1/4(SOHc / 0..1) -> Rate Transition2/1, Rate Transition1/1
  SOC_init/1 -> SOC coloumb counting1/1(SOC_init), ETA Model 1/5(SOC_init)
  Rate Transition1/1 -> SOC coloumb counting1/4(SOHc)
  SOHc_init/1 -> ETA Model 1/3(SOHc_init)
  ETA Model 1/7(SOHr / 1) -> Rate Transition/1
  ETA Model 1/1(Current / A) -> Delay/1
  ETA Model 1/5(T_sim / °C) -> SOC coloumb counting1/5(Tcell)
  SOC coloumb counting1/1(SOC) -> ETA Model 1/7(SOC_in)
  Delay/1 -> SOC coloumb counting1/3(I [A])
  Bus Creator1/1 -> ETA Model 1/8(SOH)
  Rate Transition2/1 -> Bus Creator1/1  "SOHc"
  SOHr_init/1 -> ETA Model 1/4(SOHr_init)
  ETA Model 1/6(Generated Heat / W) -> Terminator/1
  Gain/1 -> ETA Model 1/1("Current ")
  ETA Model 1/8(Power_sim / W) -> Terminator1/1
  ETA Model 1/3(SOC / 0..1) -> SOC/1
  PS-Simulink Converter/1 -> Voltage/1
  "Current / A "/1 -> Simulink-PS Converter2/1, Gain/1
  ETA Model 1/2(Voltage / V) -> Simulink-PS Converter1/1
  ETA Model 1/9(total_Ah) -> Terminator2/1
  connections:
  Controlled Current Source2/RConn2 -- Voltage Sensor1/LConn1 -- Controlled Voltage Source/LConn1
  PS-Simulink Converter/LConn1 -- Voltage Sensor1/RConn1
  Simulink-PS Converter1/RConn1 -- Controlled Voltage Source/RConn1
  Controlled Current Source2/RConn1 -- Simulink-PS Converter2/RConn1
  Cell +/RConn1 -- Controlled Current Source2/LConn1
  Controlled Voltage Source/RConn2 -- Cell -/RConn1
  Electrical Reference2/LConn1 -- Voltage Sensor1/RConn2

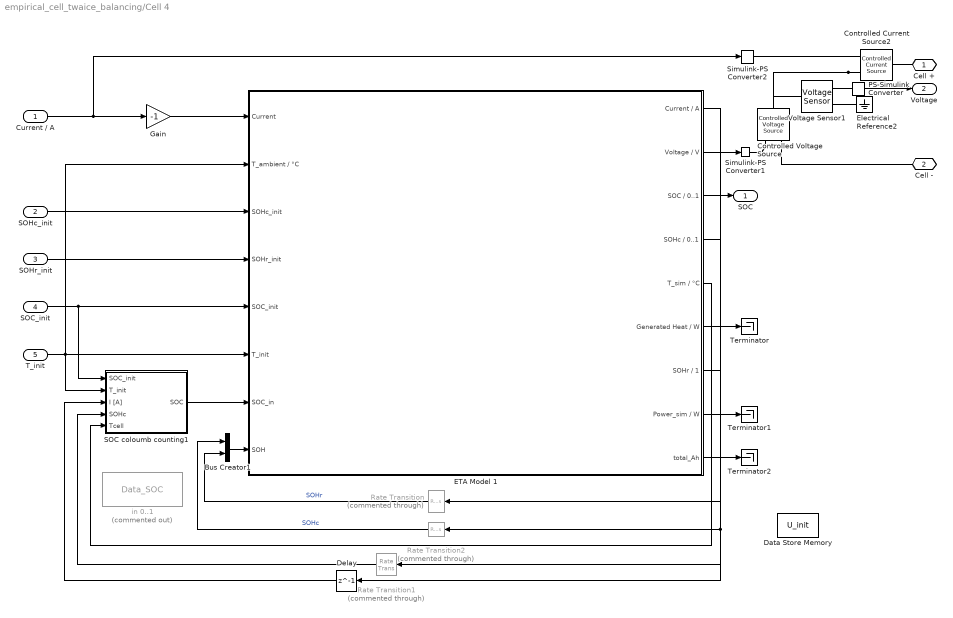
== system empirical_cell_twaice_balancing/Cell 4 ==
  "Current / A " : Inport  OutDataTypeStr=double  PortDimensions=1
  SOHc_init : Inport  Port=2
  SOHr_init : Inport  Port=3
  SOC_init : Inport  Port=4
  T_init : Inport  Port=5
  Bus Creator1 : BusCreator  Inputs=2
  Controlled Current Source2 : fl_lib/Electrical/Electrical Sources/Controlled Current Source
  Controlled Voltage Source : fl_lib/Electrical/Electrical Sources/Controlled Voltage Source
  Data Store Memory : DataStoreMemory  DataStoreName=U_init  WriteAfterWriteMsg=warning  ShowAdditionalParam=off
  Delay : Delay  DelayLength=1
  ETA Model 1 : Subsystem  mask{sfcnParam1=Ts, sfcnParam2=act, sfcnParam3=lic_no}
      mask prompts: sfcnParam1 "Ts:"; sfcnParam2 "act:"; sfcnParam3 "lic_no:"
      mask help: Simulink:masks:GenSFuncDesc_MD
      mask Help: eval('feval(''rtwprivate'',''rtwhelpview'',''rtw_sfcn_block'')');
  Electrical Reference2 : fl_lib/Electrical/Electrical Elements/Electrical Reference
  Gain : Gain  Gain=-1
  PS-Simulink Converter : nesl_utility/PS-Simulink Converter  PhysicalDomain=network_engine_domain  SubClassName=ps_output  LeftPortType=input  RightPortType=output  PseudoPeriodic=off  Frequencies=[]  VectorFormat=inherit  Unit=inherit  AffineConversion=on
  Rate Transition : RateTransition  Commented=through  InitialCondition=SOHr_init
  Rate Transition1 : RateTransition  Commented=through  InitialCondition=SOHc_init
  Rate Transition2 : RateTransition  Commented=through  InitialCondition=SOHc_init
  SOC coloumb counting1 : Subsystem  mask{sfcnParam1=Ts}
      mask prompts: sfcnParam1 "Ts:"
      mask help: Simulink:masks:GenSFuncDesc_MD
      mask Help: eval('feval(''rtwprivate'',''rtwhelpview'',''rtw_sfcn_block'')');
  Simulink-PS Converter1 : nesl_utility/Simulink-PS Converter  PhysicalDomain=network_engine_domain  SubClassName=ps_input  LeftPortType=input  RightPortType=output  PseudoPeriodic=off  Frequencies=[]  NoiseDistribution=none  NoiseParameters=[]  Unit=1  AffineConversion=on  FilteringAndDerivatives=provide  SimscapeFilterOrder=1  InputFilterTimeConstant=0.001  UdotUserProvided=0
  Simulink-PS Converter2 : nesl_utility/Simulink-PS Converter  PhysicalDomain=network_engine_domain  SubClassName=ps_input  LeftPortType=input  RightPortType=output  PseudoPeriodic=off  Frequencies=[]  NoiseDistribution=none  NoiseParameters=[]  Unit=1  AffineConversion=on  FilteringAndDerivatives=provide  SimscapeFilterOrder=1  InputFilterTimeConstant=0.001  UdotUserProvided=0
  Terminator : Terminator
  Terminator1 : Terminator
  Terminator2 : Terminator
  Voltage Sensor1 : fl_lib/Electrical/Electrical Sensors/Voltage Sensor
  in 0..1 : FromWorkspace  Commented=on  VariableName=Data_SOC  SampleTime=Ts  OutputAfterFinalValue=Setting to zero
  Cell + : PMIOPort  Side=Right
  Cell - : PMIOPort  Port=2  Side=Right
  SOC : Outport
  Voltage : Outport  Port=2
  wires:
  Rate Transition/1 -> Bus Creator1/2  "SOHr"
  T_init/1 -> ETA Model 1/2(T_ambient / °C), SOC coloumb counting1/2(T_init), ETA Model 1/6(T_init)
  ETA Model 1/4(SOHc / 0..1) -> Rate Transition2/1, Rate Transition1/1
  SOC_init/1 -> SOC coloumb counting1/1(SOC_init), ETA Model 1/5(SOC_init)
  Rate Transition1/1 -> SOC coloumb counting1/4(SOHc)
  SOHc_init/1 -> ETA Model 1/3(SOHc_init)
  ETA Model 1/7(SOHr / 1) -> Rate Transition/1
  ETA Model 1/1(Current / A) -> Delay/1
  ETA Model 1/5(T_sim / °C) -> SOC coloumb counting1/5(Tcell)
  SOC coloumb counting1/1(SOC) -> ETA Model 1/7(SOC_in)
  Delay/1 -> SOC coloumb counting1/3(I [A])
  Bus Creator1/1 -> ETA Model 1/8(SOH)
  Rate Transition2/1 -> Bus Creator1/1  "SOHc"
  SOHr_init/1 -> ETA Model 1/4(SOHr_init)
  Gain/1 -> ETA Model 1/1("Current ")
  PS-Simulink Converter/1 -> Voltage/1
  "Current / A "/1 -> Simulink-PS Converter2/1, Gain/1
  ETA Model 1/9(total_Ah) -> Terminator2/1
  ETA Model 1/3(SOC / 0..1) -> SOC/1
  ETA Model 1/2(Voltage / V) -> Simulink-PS Converter1/1
  ETA Model 1/8(Power_sim / W) -> Terminator1/1
  ETA Model 1/6(Generated Heat / W) -> Terminator/1
  connections:
  Controlled Current Source2/RConn2 -- Voltage Sensor1/LConn1 -- Controlled Voltage Source/LConn1
  Electrical Reference2/LConn1 -- Voltage Sensor1/RConn2
  Cell +/RConn1 -- Controlled Current Source2/LConn1
  Simulink-PS Converter1/RConn1 -- Controlled Voltage Source/RConn1
  Controlled Current Source2/RConn1 -- Simulink-PS Converter2/RConn1
  Controlled Voltage Source/RConn2 -- Cell -/RConn1
  PS-Simulink Converter/LConn1 -- Voltage Sensor1/RConn1

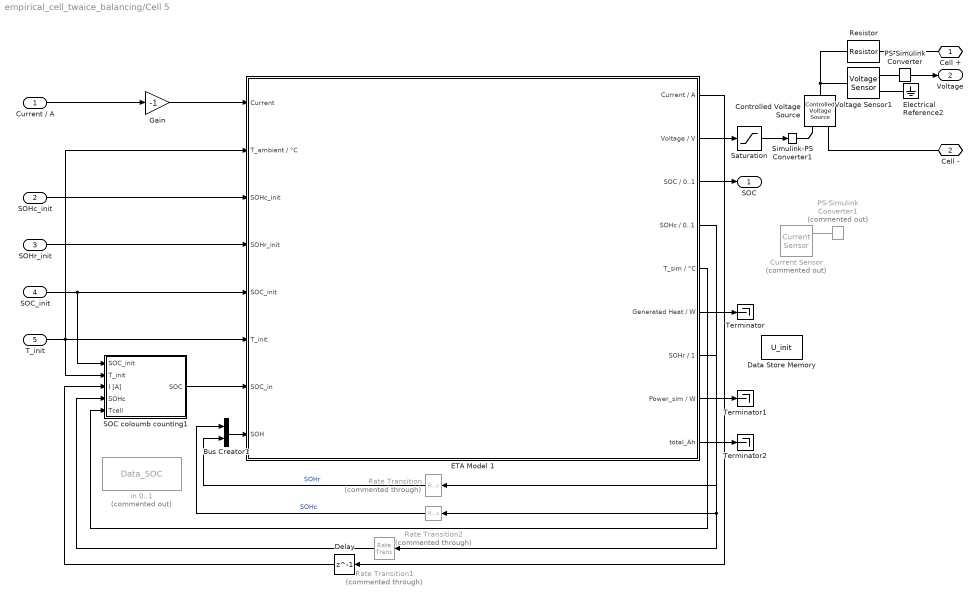
== system empirical_cell_twaice_balancing/Cell 5 ==
  "Current / A " : Inport  OutDataTypeStr=double  PortDimensions=1
  SOHc_init : Inport  Port=2
  SOHr_init : Inport  Port=3
  SOC_init : Inport  Port=4
  T_init : Inport  Port=5
  Bus Creator1 : BusCreator  Inputs=2
  Controlled Voltage Source : fl_lib/Electrical/Electrical Sources/Controlled Voltage Source
  Current Sensor : fl_lib/Electrical/Electrical Sensors/Current Sensor  Commented=on
  Data Store Memory : DataStoreMemory  DataStoreName=U_init  WriteAfterWriteMsg=warning  ShowAdditionalParam=off
  Delay : Delay  DelayLength=1
  ETA Model 1 : Subsystem  mask{sfcnParam1=Ts, sfcnParam2=act, sfcnParam3=lic_no}
      mask prompts: sfcnParam1 "Ts:"; sfcnParam2 "act:"; sfcnParam3 "lic_no:"
      mask help: Simulink:masks:GenSFuncDesc_MD
      mask Help: eval('feval(''rtwprivate'',''rtwhelpview'',''rtw_sfcn_block'')');
  Electrical Reference2 : fl_lib/Electrical/Electrical Elements/Electrical Reference
  Gain : Gain  Gain=-1
  PS-Simulink Converter : nesl_utility/PS-Simulink Converter  PhysicalDomain=network_engine_domain  SubClassName=ps_output  LeftPortType=input  RightPortType=output  PseudoPeriodic=off  Frequencies=[]  VectorFormat=inherit  Unit=inherit  AffineConversion=on
  PS-Simulink Converter1 : nesl_utility/PS-Simulink Converter  Commented=on  PhysicalDomain=network_engine_domain  SubClassName=ps_output  LeftPortType=input  RightPortType=output  PseudoPeriodic=off  Frequencies=[]  VectorFormat=inherit  Unit=inherit  AffineConversion=on
  Rate Transition : RateTransition  Commented=through  InitialCondition=SOHr_init
  Rate Transition1 : RateTransition  Commented=through  InitialCondition=SOHc_init
  Rate Transition2 : RateTransition  Commented=through  InitialCondition=SOHc_init
  Resistor : fl_lib/Electrical/Electrical Elements/Resistor  R=1 mOhm  i_specify=off  i_priority=None  i=0 A  i_nominal_specify=off  i_nominal_value=1  i_nominal_unit=A  v_specify=off  v_priority=None  v=0 V  v_nominal_specify=off  v_nominal_value=1  v_nominal_unit=V
  SOC coloumb counting1 : Subsystem  mask{sfcnParam1=Ts}
      mask prompts: sfcnParam1 "Ts:"
      mask help: Simulink:masks:GenSFuncDesc_MD
      mask Help: eval('feval(''rtwprivate'',''rtwhelpview'',''rtw_sfcn_block'')');
  Saturation : Saturate  UpperLimit=4.15  LowerLimit=2.8
  Simulink-PS Converter1 : nesl_utility/Simulink-PS Converter  PhysicalDomain=network_engine_domain  SubClassName=ps_input  LeftPortType=input  RightPortType=output  PseudoPeriodic=off  Frequencies=[]  NoiseDistribution=none  NoiseParameters=[]  Unit=1  AffineConversion=on  FilteringAndDerivatives=provide  SimscapeFilterOrder=1  InputFilterTimeConstant=0.001  UdotUserProvided=0
  Terminator : Terminator
  Terminator1 : Terminator
  Terminator2 : Terminator
  Voltage Sensor1 : fl_lib/Electrical/Electrical Sensors/Voltage Sensor
  in 0..1 : FromWorkspace  Commented=on  VariableName=Data_SOC  SampleTime=Ts  OutputAfterFinalValue=Setting to zero
  Cell + : PMIOPort  Side=Right
  Cell - : PMIOPort  Port=2  Side=Right
  SOC : Outport
  Voltage : Outport  Port=2
  wires:
  Rate Transition/1 -> Bus Creator1/2  "SOHr"
  T_init/1 -> ETA Model 1/2(T_ambient / °C), SOC coloumb counting1/2(T_init), ETA Model 1/6(T_init)
  ETA Model 1/3(SOC / 0..1) -> SOC/1
  ETA Model 1/4(SOHc / 0..1) -> Rate Transition2/1, Rate Transition1/1
  SOC_init/1 -> SOC coloumb counting1/1(SOC_init), ETA Model 1/5(SOC_init)
  Rate Transition1/1 -> SOC coloumb counting1/4(SOHc)
  SOHc_init/1 -> ETA Model 1/3(SOHc_init)
  ETA Model 1/9(total_Ah) -> Terminator2/1
  ETA Model 1/7(SOHr / 1) -> Rate Transition/1
  ETA Model 1/1(Current / A) -> Delay/1
  ETA Model 1/5(T_sim / °C) -> SOC coloumb counting1/5(Tcell)
  SOC coloumb counting1/1(SOC) -> ETA Model 1/7(SOC_in)
  ETA Model 1/8(Power_sim / W) -> Terminator1/1
  Delay/1 -> SOC coloumb counting1/3(I [A])
  Bus Creator1/1 -> ETA Model 1/8(SOH)
  Rate Transition2/1 -> Bus Creator1/1  "SOHc"
  SOHr_init/1 -> ETA Model 1/4(SOHr_init)
  ETA Model 1/6(Generated Heat / W) -> Terminator/1
  Gain/1 -> ETA Model 1/1("Current ")
  "Current / A "/1 -> Gain/1
  PS-Simulink Converter/1 -> Voltage/1
  ETA Model 1/2(Voltage / V) -> Saturation/1
  Saturation/1 -> Simulink-PS Converter1/1
  connections:
  Voltage Sensor1/LConn1 -- Resistor/LConn1 -- Controlled Voltage Source/LConn1
  Electrical Reference2/LConn1 -- Voltage Sensor1/RConn2
  PS-Simulink Converter/LConn1 -- Voltage Sensor1/RConn1
  Current Sensor/RConn1 -- PS-Simulink Converter1/LConn1
  Controlled Voltage Source/RConn2 -- Cell -/RConn1
  Simulink-PS Converter1/RConn1 -- Controlled Voltage Source/RConn1
  Cell +/RConn1 -- Resistor/RConn1
